simulink model "nonlinsim"  (R2018b)
settings: Solver=ode1  StartTime=t_start  StopTime=t_stop  FixedStep=dt  RelTol=1e-3
values from neighbouring files (symbols this model uses):
  chi0 = 0    [runsim_nonlin.m]
  chidot_max = 30*pi/180    (= 0.523598775598)    [runsim_nonlin.m]
  chidot_min = -30*pi/180    (= -0.523598775598)    [runsim_nonlin.m]
  E0 = 0    [runsim_nonlin.m]
  E01 = 0    [runsim_nonlin.m]
  intg_Ki_E = V0*sin(chi0)    [runsim_nonlin.m]
  intg_Ki_E1 = V01*sin(chi01)    [runsim_nonlin.m]
  intg_Ki_N = V0*cos(chi0)    [runsim_nonlin.m]
  intg_Ki_N1 = V01*cos(chi01)    [runsim_nonlin.m]
  Ki_E = 0    [runsim_nonlin.m]
  Ki_N = 0    [runsim_nonlin.m]
  Kp_E = 1    [runsim_nonlin.m]
  Kp_Edot = 2.5    [runsim_nonlin.m]
  Kp_N = 1    [runsim_nonlin.m]
  Kp_Ndot = 2.5    [runsim_nonlin.m]
  N0 = 0    [runsim_nonlin.m]
  N01 = 150    [runsim_nonlin.m]
  V0 = 40*mph2fps    (= 58.8)    [runsim_nonlin.m]
  V_max = 45*mph2fps    (= 66.15)    [runsim_nonlin.m]
  V_min = 0    [runsim_nonlin.m]
  Vdot_max = 0.5*g    (= 16.1)    [runsim_nonlin.m]
  Vdot_min = -0.5*g    (= -16.1)    [runsim_nonlin.m]
settings Model: Creator=suvo.ganguli  LastModifiedBy=suvo.ganguli

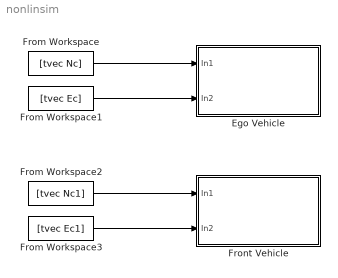
== system nonlinsim ==
  Ego Vehicle : Subsystem
  From Workspace : FromWorkspace  VariableName=[tvec Nc]  SampleTime=0
  From Workspace1 : FromWorkspace  VariableName=[tvec Ec]  SampleTime=0
  From Workspace2 : FromWorkspace  VariableName=[tvec Nc1]  SampleTime=0
  From Workspace3 : FromWorkspace  VariableName=[tvec Ec1]  SampleTime=0
  Front Vehicle : Subsystem
  wires:
  From Workspace/1 -> Ego Vehicle/1(In1)
  From Workspace1/1 -> Ego Vehicle/2(In2)
  From Workspace3/1 -> Front Vehicle/2(In2)
  From Workspace2/1 -> Front Vehicle/1(In1)

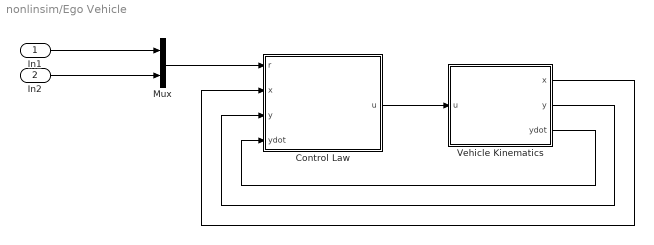
== system nonlinsim/Ego Vehicle ==
  In1 : Inport
  In2 : Inport  Port=2
  Control Law : Subsystem
  Mux : Mux  Inputs=2
  Vehicle Kinematics : Subsystem
  wires:
  In1/1 -> Mux/1
  Control Law/1(u) -> Vehicle Kinematics/1(u)
  Vehicle Kinematics/3(ydot) -> Control Law/4(ydot)
  Vehicle Kinematics/1(x) -> Control Law/2(x)
  Vehicle Kinematics/2(y) -> Control Law/3(y)
  Mux/1 -> Control Law/1(r)
  In2/1 -> Mux/2

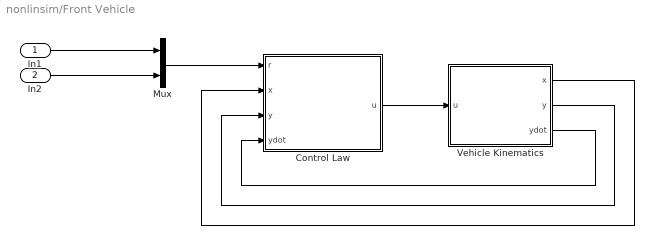
== system nonlinsim/Front Vehicle ==
  In1 : Inport
  In2 : Inport  Port=2
  Control Law : Subsystem
  Mux : Mux  Inputs=2
  Vehicle Kinematics : Subsystem
  wires:
  In2/1 -> Mux/2
  Mux/1 -> Control Law/1(r)
  Vehicle Kinematics/2(y) -> Control Law/3(y)
  Vehicle Kinematics/1(x) -> Control Law/2(x)
  Vehicle Kinematics/3(ydot) -> Control Law/4(ydot)
  Control Law/1(u) -> Vehicle Kinematics/1(u)
  In1/1 -> Mux/1

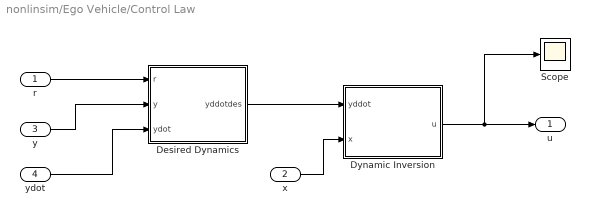
== system nonlinsim/Ego Vehicle/Control Law ==
  r : Inport
  x : Inport  Port=2
  y : Inport  Port=3
  ydot : Inport  Port=4
  Desired Dynamics : Subsystem
  Dynamic Inversion : Subsystem
  Scope : Scope
  u : Outport
  wires:
  r/1 -> Desired Dynamics/1(r)
  Desired Dynamics/1(yddotdes) -> Dynamic Inversion/1(yddot)
  Dynamic Inversion/1(u) -> Scope/1, u/1
  y/1 -> Desired Dynamics/2(y)
  x/1 -> Dynamic Inversion/2(x)
  ydot/1 -> Desired Dynamics/3(ydot)

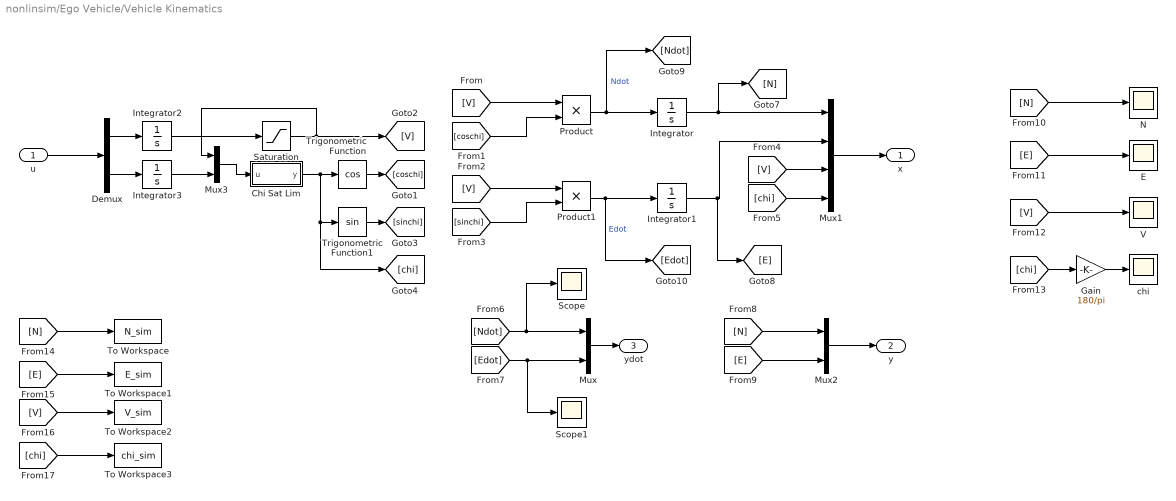
== system nonlinsim/Ego Vehicle/Vehicle Kinematics ==
  u : Inport
  Chi Sat Lim : MATLAB Function  TreatAsAtomicUnit=on
  Demux : Demux  Outputs=2
  E : Scope
  Gain : Gain  Gain=180/pi
  Integrator : Integrator  InitialCondition=N0
  Integrator1 : Integrator  InitialCondition=E0
  Integrator2 : Integrator  InitialCondition=V0
  Integrator3 : Integrator  InitialCondition=chi0
  Mux : Mux  Inputs=2
  Mux1 : Mux
  Mux2 : Mux  Inputs=2
  Mux3 : Mux  Inputs=2
  N : Scope
  Product : Product
  Product1 : Product
  Saturation : Saturate  UpperLimit=V_max  LowerLimit=V_min
  Scope : Scope
  Scope1 : Scope
  To Workspace : ToWorkspace  VariableName=N_sim  SampleTime=-1
  To Workspace1 : ToWorkspace  VariableName=E_sim  SampleTime=-1
  To Workspace2 : ToWorkspace  VariableName=V_sim  SampleTime=-1
  To Workspace3 : ToWorkspace  VariableName=chi_sim  SampleTime=-1
  Trigonometric Function : Trigonometry  Operator=cos
  Trigonometric Function1 : Trigonometry
  V : Scope
  chi : Scope
  x : Outport
  y : Outport  Port=2
  ydot : Outport  Port=3
  wires:
  [V] -> Product/1
  Integrator2/1 -> Saturation/1
  Trigonometric Function/1 -> [coschi]
  Demux/1 -> Integrator2/1
  Product/1 -> [Ndot], Integrator/1  "Ndot"
  Integrator1/1 -> [E], Mux1/2
  Integrator/1 -> [N], Mux1/1
  Demux/2 -> Integrator3/1
  [coschi] -> Product/2
  [sinchi] -> Product1/2
  [V] -> Product1/1
  Product1/1 -> [Edot], Integrator1/1  "Edot"
  Trigonometric Function1/1 -> [sinchi]
  u/1 -> Demux/1
  [V] -> Mux1/3
  [chi] -> Mux1/4
  Mux1/1 -> x/1
  Mux/1 -> ydot/1
  Mux2/1 -> y/1
  [E] -> Mux2/2
  [N] -> Mux2/1
  [Ndot] -> Scope/1, Mux/1
  [Edot] -> Scope1/1, Mux/2
  [N] -> N/1
  [E] -> E/1
  [V] -> V/1
  [chi] -> Gain/1
  Gain/1 -> chi/1
  [N] -> To Workspace/1
  [E] -> To Workspace1/1
  [V] -> To Workspace2/1
  [chi] -> To Workspace3/1
  Saturation/1 -> Mux3/1, [V]
  Integrator3/1 -> Mux3/2
  Chi Sat Lim/1(y) -> [chi], Trigonometric Function1/1, Trigonometric Function/1
  Mux3/1 -> Chi Sat Lim/1(u)

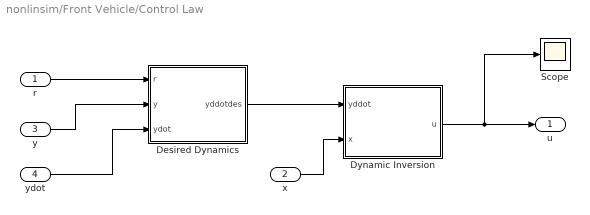
== system nonlinsim/Front Vehicle/Control Law ==
  r : Inport
  x : Inport  Port=2
  y : Inport  Port=3
  ydot : Inport  Port=4
  Desired Dynamics : Subsystem
  Dynamic Inversion : Subsystem
  Scope : Scope
  u : Outport
  wires:
  ydot/1 -> Desired Dynamics/3(ydot)
  x/1 -> Dynamic Inversion/2(x)
  y/1 -> Desired Dynamics/2(y)
  Dynamic Inversion/1(u) -> u/1, Scope/1
  Desired Dynamics/1(yddotdes) -> Dynamic Inversion/1(yddot)
  r/1 -> Desired Dynamics/1(r)

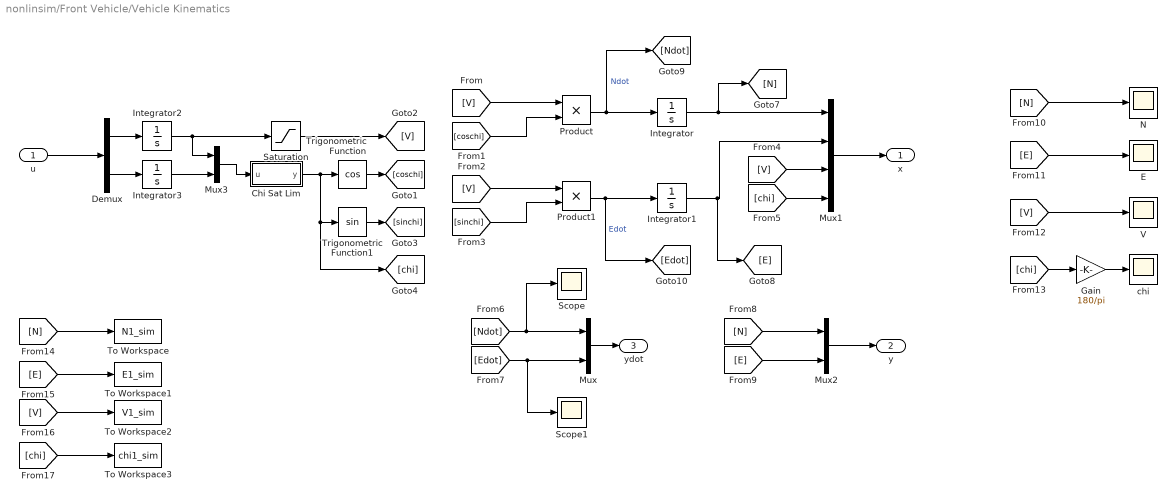
== system nonlinsim/Front Vehicle/Vehicle Kinematics ==
  u : Inport
  Chi Sat Lim : MATLAB Function  TreatAsAtomicUnit=on
  Demux : Demux  Outputs=2
  E : Scope
  Gain : Gain  Gain=180/pi
  Integrator : Integrator  InitialCondition=N01
  Integrator1 : Integrator  InitialCondition=E01
  Integrator2 : Integrator  InitialCondition=V0
  Integrator3 : Integrator  InitialCondition=chi0
  Mux : Mux  Inputs=2
  Mux1 : Mux
  Mux2 : Mux  Inputs=2
  Mux3 : Mux  Inputs=2
  N : Scope
  Product : Product
  Product1 : Product
  Saturation : Saturate  UpperLimit=V_max  LowerLimit=V_min
  Scope : Scope
  Scope1 : Scope
  To Workspace : ToWorkspace  VariableName=N1_sim  SampleTime=-1
  To Workspace1 : ToWorkspace  VariableName=E1_sim  SampleTime=-1
  To Workspace2 : ToWorkspace  VariableName=V1_sim  SampleTime=-1
  To Workspace3 : ToWorkspace  VariableName=chi1_sim  SampleTime=-1
  Trigonometric Function : Trigonometry  Operator=cos
  Trigonometric Function1 : Trigonometry
  V : Scope
  chi : Scope
  x : Outport
  y : Outport  Port=2
  ydot : Outport  Port=3
  wires:
  [chi] -> To Workspace3/1
  [V] -> To Workspace2/1
  [E] -> To Workspace1/1
  [N] -> To Workspace/1
  Gain/1 -> chi/1
  [chi] -> Gain/1
  [V] -> V/1
  [E] -> E/1
  [N] -> N/1
  [Edot] -> Mux/2, Scope1/1
  [Ndot] -> Mux/1, Scope/1
  [N] -> Mux2/1
  [E] -> Mux2/2
  Mux2/1 -> y/1
  Mux/1 -> ydot/1
  Mux1/1 -> x/1
  [chi] -> Mux1/4
  [V] -> Mux1/3
  u/1 -> Demux/1
  Product1/1 -> Integrator1/1, [Edot]  "Edot"
  [V] -> Product1/1
  [sinchi] -> Product1/2
  [coschi] -> Product/2
  Integrator/1 -> Mux1/1, [N]
  Integrator1/1 -> Mux1/2, [E]
  Product/1 -> Integrator/1, [Ndot]  "Ndot"
  [V] -> Product/1
  Integrator3/1 -> Mux3/2
  Chi Sat Lim/1(y) -> [chi], Trigonometric Function1/1, Trigonometric Function/1
  Mux3/1 -> Chi Sat Lim/1(u)
  Saturation/1 -> [V]
  Demux/1 -> Integrator2/1
  Demux/2 -> Integrator3/1
  Integrator2/1 -> Mux3/1, Saturation/1
  Trigonometric Function/1 -> [coschi]
  Trigonometric Function1/1 -> [sinchi]

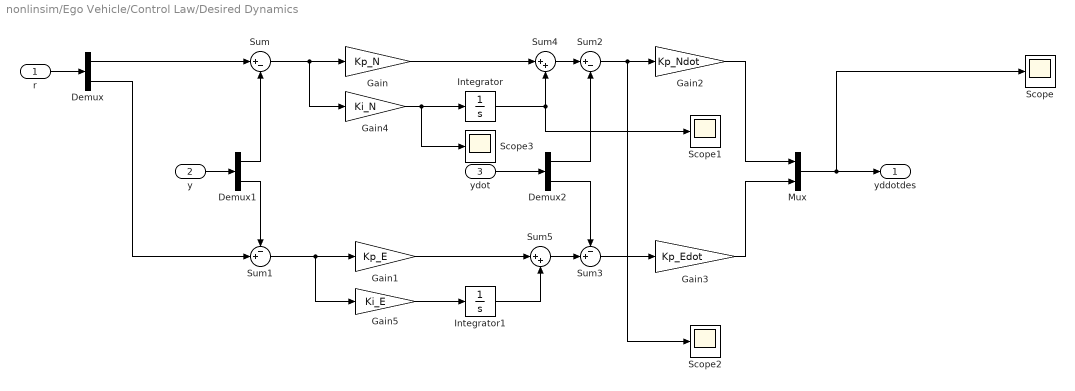
== system nonlinsim/Ego Vehicle/Control Law/Desired Dynamics ==
  r : Inport
  y : Inport  Port=2
  ydot : Inport  Port=3
  Demux : Demux  Outputs=2
  Demux1 : Demux  Outputs=2
  Demux2 : Demux  Outputs=2
  Gain : Gain  Gain=Kp_N
  Gain1 : Gain  Gain=Kp_E
  Gain2 : Gain  Gain=Kp_Ndot
  Gain3 : Gain  Gain=Kp_Edot
  Gain4 : Gain  Gain=Ki_N
  Gain5 : Gain  Gain=Ki_E
  Integrator : Integrator  InitialCondition=intg_Ki_N
  Integrator1 : Integrator  InitialCondition=intg_Ki_E
  Mux : Mux  Inputs=2
  Scope{,1..3} (4 alike) : Scope
  Sum : Sum  Inputs=|+-
  Sum1 : Sum  Inputs=-+|
  Sum2 : Sum  Inputs=|+-
  Sum3 : Sum  Inputs=-+|
  Sum4 : Sum  Inputs=|++
  Sum5 : Sum  Inputs=|++
  yddotdes : Outport
  wires:
  r/1 -> Demux/1
  y/1 -> Demux1/1
  Demux/1 -> Sum/1
  Demux1/1 -> Sum/2
  Demux1/2 -> Sum1/1
  Mux/1 -> Scope/1, yddotdes/1
  Demux/2 -> Sum1/2
  ydot/1 -> Demux2/1
  Demux2/1 -> Sum2/2
  Demux2/2 -> Sum3/1
  Sum2/1 -> Scope2/1, Gain2/1
  Sum3/1 -> Gain3/1
  Gain2/1 -> Mux/1
  Gain3/1 -> Mux/2
  Gain/1 -> Sum4/1
  Sum4/1 -> Sum2/1
  Sum/1 -> Gain4/1, Gain/1
  Integrator/1 -> Sum4/2, Scope1/1
  Gain4/1 -> Scope3/1, Integrator/1
  Gain5/1 -> Integrator1/1
  Sum1/1 -> Gain5/1, Gain1/1
  Gain1/1 -> Sum5/1
  Sum5/1 -> Sum3/2
  Integrator1/1 -> Sum5/2

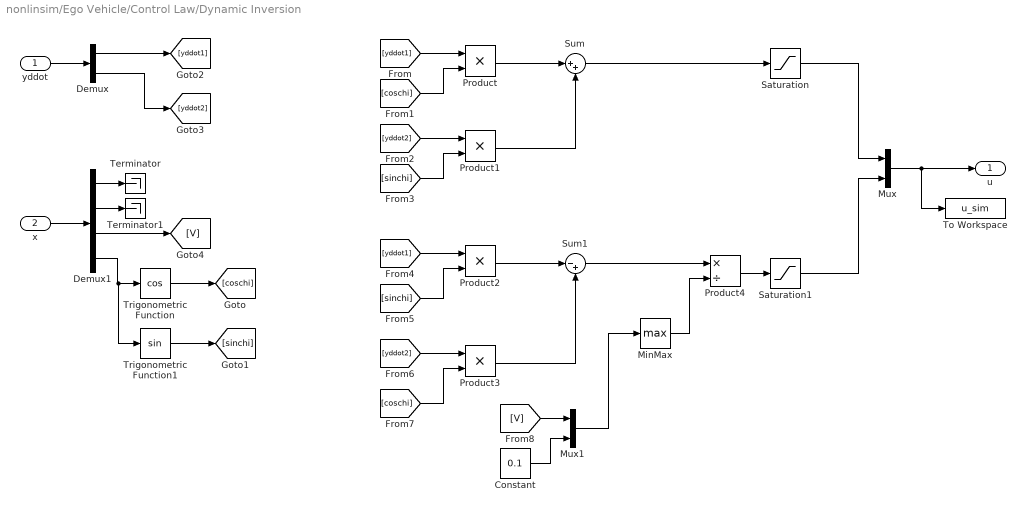
== system nonlinsim/Ego Vehicle/Control Law/Dynamic Inversion ==
  yddot : Inport
  x : Inport  Port=2
  Constant : Constant  Value=0.1
  Demux : Demux  Outputs=2
  Demux1 : Demux
  MinMax : MinMax  Function=max
  Mux : Mux  Inputs=2
  Mux1 : Mux  Inputs=2
  Product{,1..3} (4 alike) : Product
  Product4 : Product  Inputs=*/
  Saturation : Saturate  UpperLimit=Vdot_max  LowerLimit=Vdot_min
  Saturation1 : Saturate  UpperLimit=chidot_max  LowerLimit=chidot_min
  Sum : Sum  Inputs=|++
  Sum1 : Sum  Inputs=|-+
  Terminator : Terminator
  Terminator1 : Terminator
  To Workspace : ToWorkspace  VariableName=u_sim  SampleTime=-1
  Trigonometric Function : Trigonometry  Operator=cos
  Trigonometric Function1 : Trigonometry
  u : Outport
  wires:
  yddot/1 -> Demux/1
  Product/1 -> Sum/1
  Product2/1 -> Sum1/1
  Product3/1 -> Sum1/2
  Trigonometric Function/1 -> [coschi]
  Trigonometric Function1/1 -> [sinchi]
  Demux/1 -> [yddot1]
  Demux/2 -> [yddot2]
  [yddot1] -> Product/1
  [coschi] -> Product/2
  [yddot2] -> Product1/1
  [sinchi] -> Product1/2
  Product1/1 -> Sum/2
  [yddot1] -> Product2/1
  [sinchi] -> Product2/2
  [yddot2] -> Product3/1
  [coschi] -> Product3/2
  Mux/1 -> To Workspace/1, u/1
  Sum/1 -> Saturation/1
  x/1 -> Demux1/1
  Sum1/1 -> Product4/1
  Product4/1 -> Saturation1/1
  [V] -> Mux1/1
  Constant/1 -> Mux1/2
  Mux1/1 -> MinMax/1
  MinMax/1 -> Product4/2
  Demux1/1 -> Terminator/1
  Demux1/2 -> Terminator1/1
  Demux1/3 -> [V]
  Demux1/4 -> Trigonometric Function1/1, Trigonometric Function/1
  Saturation/1 -> Mux/1
  Saturation1/1 -> Mux/2

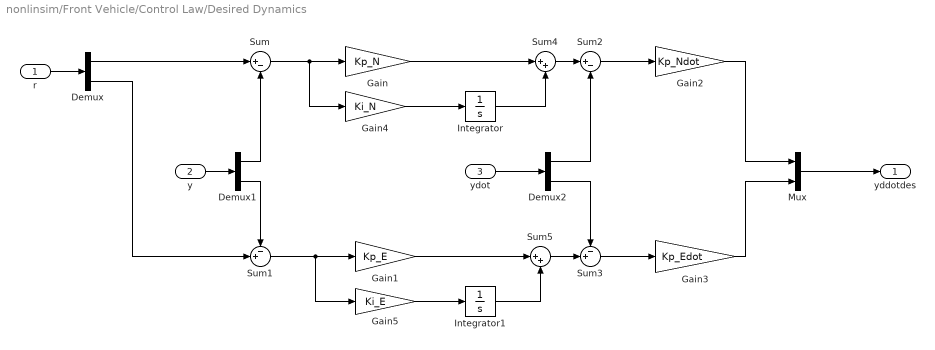
== system nonlinsim/Front Vehicle/Control Law/Desired Dynamics ==
  r : Inport
  y : Inport  Port=2
  ydot : Inport  Port=3
  Demux : Demux  Outputs=2
  Demux1 : Demux  Outputs=2
  Demux2 : Demux  Outputs=2
  Gain : Gain  Gain=Kp_N
  Gain1 : Gain  Gain=Kp_E
  Gain2 : Gain  Gain=Kp_Ndot
  Gain3 : Gain  Gain=Kp_Edot
  Gain4 : Gain  Gain=Ki_N
  Gain5 : Gain  Gain=Ki_E
  Integrator : Integrator  InitialCondition=intg_Ki_N1
  Integrator1 : Integrator  InitialCondition=intg_Ki_E1
  Mux : Mux  Inputs=2
  Sum : Sum  Inputs=|+-
  Sum1 : Sum  Inputs=-+|
  Sum2 : Sum  Inputs=|+-
  Sum3 : Sum  Inputs=-+|
  Sum4 : Sum  Inputs=|++
  Sum5 : Sum  Inputs=|++
  yddotdes : Outport
  wires:
  Integrator1/1 -> Sum5/2
  Sum5/1 -> Sum3/2
  Gain1/1 -> Sum5/1
  Sum1/1 -> Gain1/1, Gain5/1
  Gain5/1 -> Integrator1/1
  Gain4/1 -> Integrator/1
  Integrator/1 -> Sum4/2
  Sum/1 -> Gain/1, Gain4/1
  Sum4/1 -> Sum2/1
  Gain/1 -> Sum4/1
  Gain3/1 -> Mux/2
  Gain2/1 -> Mux/1
  Sum3/1 -> Gain3/1
  Sum2/1 -> Gain2/1
  Demux2/2 -> Sum3/1
  Demux2/1 -> Sum2/2
  ydot/1 -> Demux2/1
  Demux/2 -> Sum1/2
  Mux/1 -> yddotdes/1
  Demux1/2 -> Sum1/1
  Demux1/1 -> Sum/2
  Demux/1 -> Sum/1
  y/1 -> Demux1/1
  r/1 -> Demux/1

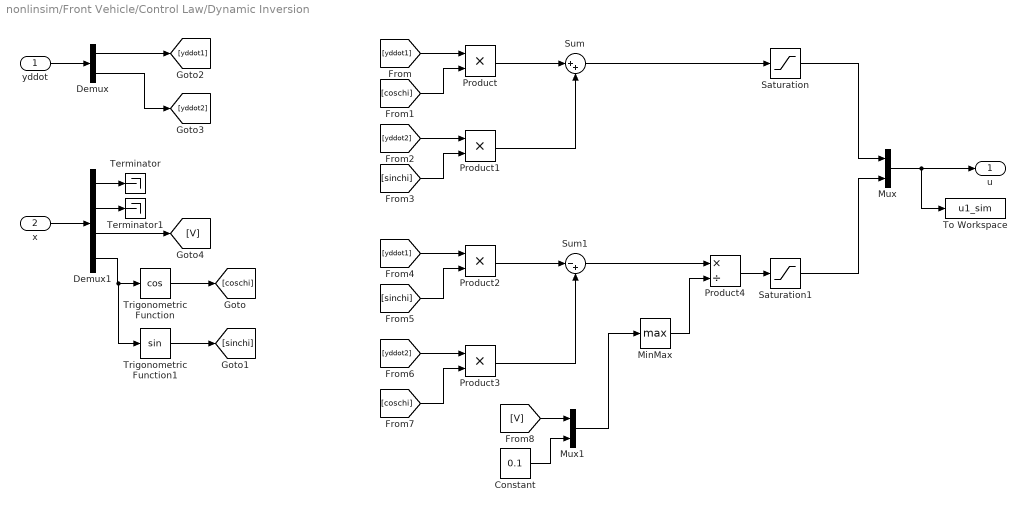
== system nonlinsim/Front Vehicle/Control Law/Dynamic Inversion ==
  yddot : Inport
  x : Inport  Port=2
  Constant : Constant  Value=0.1
  Demux : Demux  Outputs=2
  Demux1 : Demux
  MinMax : MinMax  Function=max
  Mux : Mux  Inputs=2
  Mux1 : Mux  Inputs=2
  Product{,1..3} (4 alike) : Product
  Product4 : Product  Inputs=*/
  Saturation : Saturate  UpperLimit=Vdot_max  LowerLimit=Vdot_min
  Saturation1 : Saturate  UpperLimit=chidot_max  LowerLimit=chidot_min
  Sum : Sum  Inputs=|++
  Sum1 : Sum  Inputs=|-+
  Terminator : Terminator
  Terminator1 : Terminator
  To Workspace : ToWorkspace  VariableName=u1_sim  SampleTime=-1
  Trigonometric Function : Trigonometry  Operator=cos
  Trigonometric Function1 : Trigonometry
  u : Outport
  wires:
  Saturation1/1 -> Mux/2
  Saturation/1 -> Mux/1
  Demux1/4 -> Trigonometric Function/1, Trigonometric Function1/1
  Demux1/3 -> [V]
  Demux1/2 -> Terminator1/1
  Demux1/1 -> Terminator/1
  MinMax/1 -> Product4/2
  Mux1/1 -> MinMax/1
  Constant/1 -> Mux1/2
  [V] -> Mux1/1
  Product4/1 -> Saturation1/1
  Sum1/1 -> Product4/1
  x/1 -> Demux1/1
  Sum/1 -> Saturation/1
  Mux/1 -> u/1, To Workspace/1
  [coschi] -> Product3/2
  [yddot2] -> Product3/1
  [sinchi] -> Product2/2
  [yddot1] -> Product2/1
  Product1/1 -> Sum/2
  [sinchi] -> Product1/2
  [yddot2] -> Product1/1
  [coschi] -> Product/2
  [yddot1] -> Product/1
  Demux/2 -> [yddot2]
  Demux/1 -> [yddot1]
  Trigonometric Function1/1 -> [sinchi]
  Trigonometric Function/1 -> [coschi]
  Product3/1 -> Sum1/2
  Product2/1 -> Sum1/1
  Product/1 -> Sum/1
  yddot/1 -> Demux/1

== matlab function nonlinsim/Front Vehicle/Vehicle Kinematics/Chi Sat Lim ==
  data: u input; y output
function y = fcn(u)

V = u(1);
chi = u(2);

if abs(V) < 0.1
    chi_out = 0;
else
    chi_out = chi;
end

y = chi_out;

== matlab function nonlinsim/Ego Vehicle/Vehicle Kinematics/Chi Sat Lim ==
  data: u input; y output
function y = fcn(u)

V = u(1);
chi = u(2);

if abs(V) < 0.1
    chi_out = 0;
else
    chi_out = chi;
end

y = chi_out;
